simulink model "ctc_sim"  (R2019b)
settings: Solver=VariableStepAuto  StartTime=0.0  StopTime=T  FixedStep=0.001  MaxStep=0.01  RelTol=1e-3
values from neighbouring files (symbols this model uses):
  bsc = 17    [model_data.m]
  d_r = 0.01*ones(6,1)    [model_data.m]
  Fi_b_z = [0;2/3;4/3;1/3;3/3;5/3]*pi    [model_data.m]
  ksc = 1.79e5    (= 179000)    [model_data.m]
  l_r = 0.36*ones(6,1)    [model_data.m]
  linderiv = 1    [linearize_plant.m]    (also in model_data.m = 0)
  O_lb = [0;0;0;0;0;0]    [model_data.m]
  q_d = [0.523598775598 0.523598775598 -0.713724378945 0.125327831168 0.281034901503 -0.675131532937 0.281034901503 -0.675131532937 0.523598775598 0.523598775598 -0.713724378945 0.125327831168 ... (12582 elements, 18x699)]    [ik.mat]
  qt_d = [0 0 0 0 0 0 0 0 0 0 0 0 ... (12582 elements, 18x699)]    [ik.mat]
  qtt_d = [6.28830321148e-13 -2.00728322852e-12 2.02267832113e-12 3.08516978789e-12 -6.72993285032e-12 -1.57655277981e-14 7.06082029373e-13 -2.74630882455e-12 2.48904434051e-12 -1.77039226713e-12 -3.57348306345e-12 -1.6692908872e-12 ... (12582 elements, 18x699)]    [ik.mat]
  s = out_ctc.s    [ctc_run.m]
  s_0 = s_d(:,:,1)    [ctc_run.m]    (also in iff_run.m)
  t_d = [0 0.01 0.02 0.03 0.04 0.05 0.06 0.07 0.08 0.09 0.1 0.11 ... (699 elements, 1x699)]    [ik.mat]
  v_0 = v_d(:,:,1)    [ctc_run.m]    (also in iff_run.m)
  w_lb = 0.195    [model_data.m]
  W_lb = 0.205    [model_data.m]
  w_ub = 0.195    [model_data.m]
  W_ub = 0.205    [model_data.m]
  X = fminsearch(fun,X0,opts)    [iff_diag_altopt.m]    (also in iff_single_altopt.m)
undefined symbols (not defined in the file or in its folder): Kd, Ki, Kp, Y, Z
libraries: nesl_utility x260, sm_lib x204, dspindex x30, simulink_extras x18
(part 12 of 13)

== system ctc_sim/dynamic model/rods + bases/rod 6 ==
  Mux1 : Mux  Inputs=6
  Mux2 : Mux  Inputs=6
  "O_r -> G_r" : sm_lib/Frames and Transforms/Rigid Transform  TranslationMethod=StandardAxis  TranslationStandardOffset=l_r(r)/2  TranslationLengthUnit=m  TranslationStandardAxis=-Z  TranslationCartesianOffset=[0 0 0]  TranslationROffset=0  TranslationROffsetUnits=m  TranslationZOffset=0  TranslationZOffsetUnits=m  TranslationThetaOffset=0  TranslationThetaOffsetUnits=deg  RotationMethod=None  RotationAngleUnits=deg  RotationStandardAxis=+Z  RotationAngle=0.0  RotationArbitraryAxis=[0 0 1]  FollAlignAxisA=+X  BaseAlignAxisA=+Y  FollAlignAxisB=+Y  BaseAlignAxisB=+Z  RotationSequenceAxes=FollowerAxes  RotationSequence=XYX  RotationSequenceAngles=[0 0 0]  RotationSequenceAnglesUnits=deg  RotationMatrix=[1 0 0; 0 1 0; 0 0 1]
  "O_r -> H_r" : sm_lib/Frames and Transforms/Rigid Transform  TranslationMethod=StandardAxis  TranslationStandardOffset=l_r(r)/2  TranslationLengthUnit=m  TranslationStandardAxis=+Z  TranslationCartesianOffset=[0 0 0]  TranslationROffset=0  TranslationROffsetUnits=m  TranslationZOffset=0  TranslationZOffsetUnits=m  TranslationThetaOffset=0  TranslationThetaOffsetUnits=deg  RotationMethod=None  RotationAngleUnits=deg  RotationStandardAxis=+Z  RotationAngle=0.0  RotationArbitraryAxis=[0 0 1]  FollAlignAxisA=+X  BaseAlignAxisA=+Y  FollAlignAxisB=+Y  BaseAlignAxisB=+Z  RotationSequenceAxes=FollowerAxes  RotationSequence=XYX  RotationSequenceAngles=[0 0 0]  RotationSequenceAnglesUnits=deg  RotationMatrix=[1 0 0; 0 1 0; 0 0 1]
  PS-Simulink Converter : nesl_utility/PS-Simulink Converter  PhysicalDomain=network_engine_domain  SubClassName=ps_output  LeftPortType=input  RightPortType=output  PseudoPeriodic=off  Frequencies=[]  Unit=m  AffineConversion=off
  PS-Simulink Converter1 : nesl_utility/PS-Simulink Converter  PhysicalDomain=network_engine_domain  SubClassName=ps_output  LeftPortType=input  RightPortType=output  PseudoPeriodic=off  Frequencies=[]  Unit=m  AffineConversion=off
  PS-Simulink Converter10 : nesl_utility/PS-Simulink Converter  PhysicalDomain=network_engine_domain  SubClassName=ps_output  LeftPortType=input  RightPortType=output  PseudoPeriodic=off  Frequencies=[]  Unit=m/s  AffineConversion=off
  PS-Simulink Converter11 : nesl_utility/PS-Simulink Converter  PhysicalDomain=network_engine_domain  SubClassName=ps_output  LeftPortType=input  RightPortType=output  PseudoPeriodic=off  Frequencies=[]  Unit=rad/s  AffineConversion=off
  PS-Simulink Converter12 : nesl_utility/PS-Simulink Converter  PhysicalDomain=network_engine_domain  SubClassName=ps_output  LeftPortType=input  RightPortType=output  PseudoPeriodic=off  Frequencies=[]  Unit=rad/s  AffineConversion=off
  PS-Simulink Converter13 : nesl_utility/PS-Simulink Converter  PhysicalDomain=network_engine_domain  SubClassName=ps_output  LeftPortType=input  RightPortType=output  PseudoPeriodic=off  Frequencies=[]  Unit=rad/s  AffineConversion=off
  PS-Simulink Converter2 : nesl_utility/PS-Simulink Converter  PhysicalDomain=network_engine_domain  SubClassName=ps_output  LeftPortType=input  RightPortType=output  PseudoPeriodic=off  Frequencies=[]  Unit=m  AffineConversion=off
  PS-Simulink Converter3 : nesl_utility/PS-Simulink Converter  PhysicalDomain=network_engine_domain  SubClassName=ps_output  LeftPortType=input  RightPortType=output  PseudoPeriodic=off  Frequencies=[]  Unit=rad  AffineConversion=off
  PS-Simulink Converter5 : nesl_utility/PS-Simulink Converter  PhysicalDomain=network_engine_domain  SubClassName=ps_output  LeftPortType=input  RightPortType=output  PseudoPeriodic=off  Frequencies=[]  Unit=rad  AffineConversion=off
  PS-Simulink Converter7 : nesl_utility/PS-Simulink Converter  PhysicalDomain=network_engine_domain  SubClassName=ps_output  LeftPortType=input  RightPortType=output  PseudoPeriodic=off  Frequencies=[]  Unit=rad  AffineConversion=off
  PS-Simulink Converter8 : nesl_utility/PS-Simulink Converter  PhysicalDomain=network_engine_domain  SubClassName=ps_output  LeftPortType=input  RightPortType=output  PseudoPeriodic=off  Frequencies=[]  Unit=m/s  AffineConversion=off
  PS-Simulink Converter9 : nesl_utility/PS-Simulink Converter  PhysicalDomain=network_engine_domain  SubClassName=ps_output  LeftPortType=input  RightPortType=output  PseudoPeriodic=off  Frequencies=[]  Unit=m/s  AffineConversion=off
  body_r : sm_lib/Body Elements/Cylindrical Solid  GraphicAmbientColor=[0.15 0.15 0.15 1.0]  BasedOnType=Density  CenterOfMass=[0 0 0]  CenterOfMassUnits=m  GraphicDiffuseColor=model_color  CylinderLength=l_r(r)  CylinderLengthUnits=m  CylinderRadius=d_r(r)/2  CylinderRadiusUnits=m  Density=Ro_r  DensityUnits=kg/m^3  DoExposeReferenceFrame=on  GraphicEmissiveColor=[0.0 0.0 0.0 1.0]  ExportEntireGeometry=off  SerializedFrames=<Frames/>  MarkerShape=Sphere  MarkerSize=10  GraphicType=FromGeometry  InertiaType=CalculateFromGeometry  Mass=1  MassUnits=kg  MomentsOfInertia=[1 1 1]  MomentsOfInertiaUnits=kg*m^2  GraphicOpacity=model_opacity  ProductsOfInertia=[0 0 0]  ProductsOfInertiaUnits=kg*m^2  GraphicShininess=75  GraphicSpecularColor=[0.5 0.5 0.5 1.0]  GraphicVisPropType=SimpleVisualProperties
  "wf -> O_r" : sm_lib/Joints/Bushing Joint  JointMode=Normal  SenseConstraintForce=off  SenseConstraintForceX=off  SenseConstraintForceY=off  SenseConstraintForceZ=off  SenseConstraintTorque=off  SenseConstraintTorqueX=off  SenseConstraintTorqueY=off  SenseConstraintTorqueZ=off  SenseTotalForce=off  SenseTotalForceX=off  SenseTotalForceY=off  SenseTotalForceZ=off  SenseTotalTorque=off  SenseTotalTorqueX=off  SenseTotalTorqueY=off  SenseTotalTorqueZ=off  CompositeWrenchDir=FollowerOnBase  CompositeWrenchFrame=BaseFrame  PxEquilibriumPosition=0  PxEquilibriumPositionUnits=m  PxSpringStiffness=0  PxSpringStiffnessUnits=N/m  PxDampingCoefficient=0  PxDampingCoefficientUnits=N/(m/s)  PxTorqueActuationMode=NoTorque  PxMotionActuationMode=ComputedMotion  PxSensePosition=on  PxSenseVelocity=on  PxSenseAcceleration=off  PxSenseTorqueForce=off  PxSenseLowerLimitTorqueForce=off  PxSenseUpperLimitTorqueForce=off  PxLowerLimitSpecify=off  PxLowerLimitBound=-1  PxLowerLimitBoundUnits=m  PxLowerLimitStiffness=1e6  PxLowerLimitStiffnessUnits=N/m  PxLowerLimitDamping=1e3  PxLowerLimitDampingUnits=N/(m/s)  PxLowerLimitTransitionRegionWidth=1e-4  PxLowerLimitTransitionRegionWidthUnits=m  PxUpperLimitSpecify=off  PxUpperLimitBound=1  PxUpperLimitBoundUnits=m  PxUpperLimitStiffness=1e6  PxUpperLimitStiffnessUnits=N/m  PxUpperLimitDamping=1e3  PxUpperLimitDampingUnits=N/(m/s)  PxUpperLimitTransitionRegionWidth=1e-4  PxUpperLimitTransitionRegionWidthUnits=m  PxPositionTargetSpecify=on  PxPositionTargetPriority=High  PxPositionTargetValue=s_r_0(1,r)  PxPositionTargetValueUnits=m  PxVelocityTargetSpecify=on  PxVelocityTargetPriority=High  PxVelocityTargetValue=v_r_0(1,r)  PxVelocityTargetValueUnits=m/s  PyEquilibriumPosition=0  PyEquilibriumPositionUnits=m  PySpringStiffness=0  PySpringStiffnessUnits=N/m  PyDampingCoefficient=0  PyDampingCoefficientUnits=N/(m/s)  PyTorqueActuationMode=NoTorque  PyMotionActuationMode=ComputedMotion  PySensePosition=on  PySenseVelocity=on  PySenseAcceleration=off  PySenseTorqueForce=off  PySenseLowerLimitTorqueForce=off  PySenseUpperLimitTorqueForce=off  PyLowerLimitSpecify=off  PyLowerLimitBound=-1  PyLowerLimitBoundUnits=m  PyLowerLimitStiffness=1e6  PyLowerLimitStiffnessUnits=N/m  PyLowerLimitDamping=1e3  PyLowerLimitDampingUnits=N/(m/s)  PyLowerLimitTransitionRegionWidth=1e-4  PyLowerLimitTransitionRegionWidthUnits=m  PyUpperLimitSpecify=off  PyUpperLimitBound=1  PyUpperLimitBoundUnits=m  PyUpperLimitStiffness=1e6  PyUpperLimitStiffnessUnits=N/m  PyUpperLimitDamping=1e3  PyUpperLimitDampingUnits=N/(m/s)  PyUpperLimitTransitionRegionWidth=1e-4  PyUpperLimitTransitionRegionWidthUnits=m  PyPositionTargetSpecify=on  PyPositionTargetPriority=High  PyPositionTargetValue=s_r_0(2,r)  PyPositionTargetValueUnits=m  PyVelocityTargetSpecify=on  PyVelocityTargetPriority=High  PyVelocityTargetValue=v_r_0(2,r)  PyVelocityTargetValueUnits=m/s  PzEquilibriumPosition=0  PzEquilibriumPositionUnits=m  PzSpringStiffness=0  PzSpringStiffnessUnits=N/m  PzDampingCoefficient=0  PzDampingCoefficientUnits=N/(m/s)  PzTorqueActuationMode=NoTorque  PzMotionActuationMode=ComputedMotion  PzSensePosition=on  PzSenseVelocity=on  PzSenseAcceleration=off  PzSenseTorqueForce=off  PzSenseLowerLimitTorqueForce=off  PzSenseUpperLimitTorqueForce=off  PzLowerLimitSpecify=off  PzLowerLimitBound=-1  PzLowerLimitBoundUnits=m  PzLowerLimitStiffness=1e6  PzLowerLimitStiffnessUnits=N/m  PzLowerLimitDamping=1e3  PzLowerLimitDampingUnits=N/(m/s)  PzLowerLimitTransitionRegionWidth=1e-4  PzLowerLimitTransitionRegionWidthUnits=m  PzUpperLimitSpecify=off  PzUpperLimitBound=1  PzUpperLimitBoundUnits=m  PzUpperLimitStiffness=1e6  PzUpperLimitStiffnessUnits=N/m  PzUpperLimitDamping=1e3  PzUpperLimitDampingUnits=N/(m/s)  PzUpperLimitTransitionRegionWidth=1e-4  PzUpperLimitTransitionRegionWidthUnits=m  PzPositionTargetSpecify=on  PzPositionTargetPriority=High  PzPositionTargetValue=s_r_0(3,r)  PzPositionTargetValueUnits=m  PzVelocityTargetSpecify=on  PzVelocityTargetPriority=High  PzVelocityTargetValue=v_r_0(3,r)  PzVelocityTargetValueUnits=m/s  RxEquilibriumPosition=0  RxEquilibriumPositionUnits=deg  RxSpringStiffness=0  RxSpringStiffnessUnits=N*m/deg  RxDampingCoefficient=0  RxDampingCoefficientUnits=N*m/(deg/s)  RxTorqueActuationMode=NoTorque  RxMotionActuationMode=ComputedMotion  RxSensePosition=on  RxSenseVelocity=on  RxSenseAcceleration=off  RxSenseTorqueForce=off  RxSenseLowerLimitTorqueForce=off  RxSenseUpperLimitTorqueForce=off  RxLowerLimitSpecify=off  RxLowerLimitBound=-90  RxLowerLimitBoundUnits=deg  RxLowerLimitStiffness=1e4  RxLowerLimitStiffnessUnits=N*m/deg  RxLowerLimitDamping=10  RxLowerLimitDampingUnits=N*m/(deg/s)  RxLowerLimitTransitionRegionWidth=0.1  RxLowerLimitTransitionRegionWidthUnits=deg  RxUpperLimitSpecify=off  RxUpperLimitBound=90  RxUpperLimitBoundUnits=deg  RxUpperLimitStiffness=1e4  RxUpperLimitStiffnessUnits=N*m/deg  RxUpperLimitDamping=10  RxUpperLimitDampingUnits=N*m/(deg/s)  RxUpperLimitTransitionRegionWidth=0.1  RxUpperLimitTransitionRegionWidthUnits=deg  RxPositionTargetSpecify=on  RxPositionTargetPriority=High  RxPositionTargetValue=s_r_0(4,r)  RxPositionTargetValueUnits=rad  RxVelocityTargetSpecify=on  RxVelocityTargetPriority=High  RxVelocityTargetValue=v_r_0(4,r)  RxVelocityTargetValueUnits=rad/s  RyEquilibriumPosition=0  RyEquilibriumPositionUnits=deg  RySpringStiffness=0  RySpringStiffnessUnits=N*m/deg  RyDampingCoefficient=0  RyDampingCoefficientUnits=N*m/(deg/s)  RyTorqueActuationMode=NoTorque  RyMotionActuationMode=ComputedMotion  RySensePosition=on  RySenseVelocity=on  RySenseAcceleration=off  RySenseTorqueForce=off  RySenseLowerLimitTorqueForce=off  RySenseUpperLimitTorqueForce=off  RyLowerLimitSpecify=off  RyLowerLimitBound=-90  RyLowerLimitBoundUnits=deg  RyLowerLimitStiffness=1e4  RyLowerLimitStiffnessUnits=N*m/deg  RyLowerLimitDamping=10  RyLowerLimitDampingUnits=N*m/(deg/s)  RyLowerLimitTransitionRegionWidth=0.1  RyLowerLimitTransitionRegionWidthUnits=deg  RyUpperLimitSpecify=off  RyUpperLimitBound=90  RyUpperLimitBoundUnits=deg  RyUpperLimitStiffness=1e4  RyUpperLimitStiffnessUnits=N*m/deg  RyUpperLimitDamping=10  RyUpperLimitDampingUnits=N*m/(deg/s)  RyUpperLimitTransitionRegionWidth=0.1  RyUpperLimitTransitionRegionWidthUnits=deg  RyPositionTargetSpecify=on  RyPositionTargetPriority=High  RyPositionTargetValue=s_r_0(5,r)  RyPositionTargetValueUnits=rad  RyVelocityTargetSpecify=on  RyVelocityTargetPriority=High  RyVelocityTargetValue=v_r_0(5,r)  RyVelocityTargetValueUnits=rad/s  RzEquilibriumPosition=0  RzEquilibriumPositionUnits=deg  RzSpringStiffness=0  RzSpringStiffnessUnits=N*m/deg  RzDampingCoefficient=0  RzDampingCoefficientUnits=N*m/(deg/s)  RzTorqueActuationMode=NoTorque  RzMotionActuationMode=ComputedMotion  RzSensePosition=on  RzSenseVelocity=on  RzSenseAcceleration=off  RzSenseTorqueForce=off  RzSenseLowerLimitTorqueForce=off  RzSenseUpperLimitTorqueForce=off  RzLowerLimitSpecify=off  RzLowerLimitBound=-90  RzLowerLimitBoundUnits=deg  RzLowerLimitStiffness=1e4  RzLowerLimitStiffnessUnits=N*m/deg  RzLowerLimitDamping=10  RzLowerLimitDampingUnits=N*m/(deg/s)  RzLowerLimitTransitionRegionWidth=0.1  RzLowerLimitTransitionRegionWidthUnits=deg  RzUpperLimitSpecify=off  RzUpperLimitBound=90  RzUpperLimitBoundUnits=deg  RzUpperLimitStiffness=1e4  RzUpperLimitStiffnessUnits=N*m/deg  RzUpperLimitDamping=10  RzUpperLimitDampingUnits=N*m/(deg/s)  RzUpperLimitTransitionRegionWidth=0.1  RzUpperLimitTransitionRegionWidthUnits=deg  RzPositionTargetSpecify=on  RzPositionTargetPriority=High  RzPositionTargetValue=s_r_0(6,r)  RzPositionTargetValueUnits=rad  RzVelocityTargetSpecify=on  RzVelocityTargetPriority=High  RzVelocityTargetValue=v_r_0(6,r)  RzVelocityTargetValueUnits=rad/s
      settings: SourceProductName=Simscape Multibody
  wf : PMIOPort  Side=Left
  G_r : PMIOPort  Port=2  Side=Right
  H_r : PMIOPort  Port=3  Side=Left
  s_r : Outport
  v_r : Outport  Port=2
  wires:
  Mux1/1 -> s_r/1
  PS-Simulink Converter/1 -> Mux1/1
  PS-Simulink Converter1/1 -> Mux1/2
  PS-Simulink Converter2/1 -> Mux1/3
  PS-Simulink Converter3/1 -> Mux1/4
  PS-Simulink Converter5/1 -> Mux1/5
  PS-Simulink Converter7/1 -> Mux1/6
  Mux2/1 -> v_r/1
  PS-Simulink Converter8/1 -> Mux2/1
  PS-Simulink Converter9/1 -> Mux2/2
  PS-Simulink Converter10/1 -> Mux2/3
  PS-Simulink Converter11/1 -> Mux2/4
  PS-Simulink Converter12/1 -> Mux2/5
  PS-Simulink Converter13/1 -> Mux2/6
  connections:
  "wf -> O_r"/LConn1 -- wf/RConn1
  "O_r -> G_r"/LConn1 -- body_r/RConn1 -- "wf -> O_r"/RConn1 -- "O_r -> H_r"/LConn1
  H_r/RConn1 -- "O_r -> H_r"/RConn1
  G_r/RConn1 -- "O_r -> G_r"/RConn1
  PS-Simulink Converter/LConn1 -- "wf -> O_r"/RConn2
  PS-Simulink Converter1/LConn1 -- "wf -> O_r"/RConn4
  PS-Simulink Converter2/LConn1 -- "wf -> O_r"/RConn6
  "wf -> O_r"/RConn8 -- PS-Simulink Converter3/LConn1
  PS-Simulink Converter8/LConn1 -- "wf -> O_r"/RConn3
  PS-Simulink Converter9/LConn1 -- "wf -> O_r"/RConn5
  PS-Simulink Converter10/LConn1 -- "wf -> O_r"/RConn7
  PS-Simulink Converter11/LConn1 -- "wf -> O_r"/RConn9
  PS-Simulink Converter13/LConn1 -- "wf -> O_r"/RConn13
  "wf -> O_r"/RConn12 -- PS-Simulink Converter7/LConn1
  PS-Simulink Converter12/LConn1 -- "wf -> O_r"/RConn11
  "wf -> O_r"/RConn10 -- PS-Simulink Converter5/LConn1

== system ctc_sim/dynamic model/rods + bases/upper base ==
  Mux1 : Mux  Inputs=6
  Mux2 : Mux  Inputs=6
  "O_ub -> H_4" : Subsystem
  "O_ub -> H_5" : Subsystem
  "O_ub -> H_6" : Subsystem
  PS-Simulink Converter : nesl_utility/PS-Simulink Converter  PhysicalDomain=network_engine_domain  SubClassName=ps_output  LeftPortType=input  RightPortType=output  PseudoPeriodic=off  Frequencies=[]  Unit=m  AffineConversion=off
  PS-Simulink Converter10 : nesl_utility/PS-Simulink Converter  PhysicalDomain=network_engine_domain  SubClassName=ps_output  LeftPortType=input  RightPortType=output  PseudoPeriodic=off  Frequencies=[]  Unit=rad  AffineConversion=off
  PS-Simulink Converter12 : nesl_utility/PS-Simulink Converter  PhysicalDomain=network_engine_domain  SubClassName=ps_output  LeftPortType=input  RightPortType=output  PseudoPeriodic=off  Frequencies=[]  Unit=m/s  AffineConversion=off
  PS-Simulink Converter13 : nesl_utility/PS-Simulink Converter  PhysicalDomain=network_engine_domain  SubClassName=ps_output  LeftPortType=input  RightPortType=output  PseudoPeriodic=off  Frequencies=[]  Unit=m/s  AffineConversion=off
  PS-Simulink Converter14 : nesl_utility/PS-Simulink Converter  PhysicalDomain=network_engine_domain  SubClassName=ps_output  LeftPortType=input  RightPortType=output  PseudoPeriodic=off  Frequencies=[]  Unit=m/s  AffineConversion=off
  PS-Simulink Converter15 : nesl_utility/PS-Simulink Converter  PhysicalDomain=network_engine_domain  SubClassName=ps_output  LeftPortType=input  RightPortType=output  PseudoPeriodic=off  Frequencies=[]  Unit=rad/s  AffineConversion=off
  PS-Simulink Converter16 : nesl_utility/PS-Simulink Converter  PhysicalDomain=network_engine_domain  SubClassName=ps_output  LeftPortType=input  RightPortType=output  PseudoPeriodic=off  Frequencies=[]  Unit=rad/s  AffineConversion=off
  PS-Simulink Converter17 : nesl_utility/PS-Simulink Converter  PhysicalDomain=network_engine_domain  SubClassName=ps_output  LeftPortType=input  RightPortType=output  PseudoPeriodic=off  Frequencies=[]  Unit=rad/s  AffineConversion=off
  PS-Simulink Converter2 : nesl_utility/PS-Simulink Converter  PhysicalDomain=network_engine_domain  SubClassName=ps_output  LeftPortType=input  RightPortType=output  PseudoPeriodic=off  Frequencies=[]  Unit=m  AffineConversion=off
  PS-Simulink Converter4 : nesl_utility/PS-Simulink Converter  PhysicalDomain=network_engine_domain  SubClassName=ps_output  LeftPortType=input  RightPortType=output  PseudoPeriodic=off  Frequencies=[]  Unit=m  AffineConversion=off
  PS-Simulink Converter6 : nesl_utility/PS-Simulink Converter  PhysicalDomain=network_engine_domain  SubClassName=ps_output  LeftPortType=input  RightPortType=output  PseudoPeriodic=off  Frequencies=[]  Unit=rad  AffineConversion=off
  PS-Simulink Converter8 : nesl_utility/PS-Simulink Converter  PhysicalDomain=network_engine_domain  SubClassName=ps_output  LeftPortType=input  RightPortType=output  PseudoPeriodic=off  Frequencies=[]  Unit=rad  AffineConversion=off
  body_ub : sm_lib/Body Elements/Extruded Solid  GraphicAmbientColor=[0.15 0.15 0.15 1.0]  BasedOnType=Density  CenterOfMass=[0 0 0]  CenterOfMassUnits=m  GraphicDiffuseColor=model_color  ExtrusionCrossSection=[1 1; -1 1; -1 -1; 1 -1]  ExtrusionCrossSectionUnits=m  Density=Ro_ub  DensityUnits=kg/m^3  DoExposeReferenceFrame=on  GraphicEmissiveColor=[0.0 0.0 0.0 1.0]  ExportEntireGeometry=off  ExtrusionLength=t_ub  ExtrusionLengthUnits=m  ExtrusionType=Regular  SerializedFrames=<Frames/>  MarkerShape=Sphere  MarkerSize=10  GraphicType=FromGeometry  InertiaType=CalculateFromGeometry  Mass=1  MassUnits=kg  MomentsOfInertia=[1 1 1]  MomentsOfInertiaUnits=kg*m^2  PolygonNumSides=6  GraphicOpacity=model_opacity  PolygonOuterRadius=(W_ub/2)/cosd(30)  PolygonOuterRadiusUnits=m  ProductsOfInertia=[0 0 0]  ProductsOfInertiaUnits=kg*m^2  GraphicShininess=75  GraphicSpecularColor=[0.5 0.5 0.5 1.0]  GraphicVisPropType=SimpleVisualProperties
      settings: SourceProductName=Simscape Multibody
  "wf -> O_ub" : sm_lib/Joints/Bushing Joint  JointMode=Normal  SenseConstraintForce=off  SenseConstraintForceX=off  SenseConstraintForceY=off  SenseConstraintForceZ=off  SenseConstraintTorque=off  SenseConstraintTorqueX=off  SenseConstraintTorqueY=off  SenseConstraintTorqueZ=off  SenseTotalForce=off  SenseTotalForceX=off  SenseTotalForceY=off  SenseTotalForceZ=off  SenseTotalTorque=off  SenseTotalTorqueX=off  SenseTotalTorqueY=off  SenseTotalTorqueZ=off  CompositeWrenchDir=FollowerOnBase  CompositeWrenchFrame=BaseFrame  PxEquilibriumPosition=0  PxEquilibriumPositionUnits=m  PxSpringStiffness=0  PxSpringStiffnessUnits=N/m  PxDampingCoefficient=0  PxDampingCoefficientUnits=N/(m/s)  PxTorqueActuationMode=NoTorque  PxMotionActuationMode=ComputedMotion  PxSensePosition=on  PxSenseVelocity=on  PxSenseAcceleration=off  PxSenseTorqueForce=off  PxSenseLowerLimitTorqueForce=off  PxSenseUpperLimitTorqueForce=off  PxLowerLimitSpecify=off  PxLowerLimitBound=-1  PxLowerLimitBoundUnits=m  PxLowerLimitStiffness=1e6  PxLowerLimitStiffnessUnits=N/m  PxLowerLimitDamping=1e3  PxLowerLimitDampingUnits=N/(m/s)  PxLowerLimitTransitionRegionWidth=1e-4  PxLowerLimitTransitionRegionWidthUnits=m  PxUpperLimitSpecify=off  PxUpperLimitBound=1  PxUpperLimitBoundUnits=m  PxUpperLimitStiffness=1e6  PxUpperLimitStiffnessUnits=N/m  PxUpperLimitDamping=1e3  PxUpperLimitDampingUnits=N/(m/s)  PxUpperLimitTransitionRegionWidth=1e-4  PxUpperLimitTransitionRegionWidthUnits=m  PxPositionTargetSpecify=on  PxPositionTargetPriority=High  PxPositionTargetValue=s_ub_0(1,1)  PxPositionTargetValueUnits=m  PxVelocityTargetSpecify=on  PxVelocityTargetPriority=High  PxVelocityTargetValue=v_ub_0(1,1)  PxVelocityTargetValueUnits=m/s  PyEquilibriumPosition=0  PyEquilibriumPositionUnits=m  PySpringStiffness=0  PySpringStiffnessUnits=N/m  PyDampingCoefficient=0  PyDampingCoefficientUnits=N/(m/s)  PyTorqueActuationMode=NoTorque  PyMotionActuationMode=ComputedMotion  PySensePosition=on  PySenseVelocity=on  PySenseAcceleration=off  PySenseTorqueForce=off  PySenseLowerLimitTorqueForce=off  PySenseUpperLimitTorqueForce=off  PyLowerLimitSpecify=off  PyLowerLimitBound=-1  PyLowerLimitBoundUnits=m  PyLowerLimitStiffness=1e6  PyLowerLimitStiffnessUnits=N/m  PyLowerLimitDamping=1e3  PyLowerLimitDampingUnits=N/(m/s)  PyLowerLimitTransitionRegionWidth=1e-4  PyLowerLimitTransitionRegionWidthUnits=m  PyUpperLimitSpecify=off  PyUpperLimitBound=1  PyUpperLimitBoundUnits=m  PyUpperLimitStiffness=1e6  PyUpperLimitStiffnessUnits=N/m  PyUpperLimitDamping=1e3  PyUpperLimitDampingUnits=N/(m/s)  PyUpperLimitTransitionRegionWidth=1e-4  PyUpperLimitTransitionRegionWidthUnits=m  PyPositionTargetSpecify=on  PyPositionTargetPriority=High  PyPositionTargetValue=s_ub_0(2,1)  PyPositionTargetValueUnits=m  PyVelocityTargetSpecify=on  PyVelocityTargetPriority=High  PyVelocityTargetValue=v_ub_0(2,1)  PyVelocityTargetValueUnits=m/s  PzEquilibriumPosition=0  PzEquilibriumPositionUnits=m  PzSpringStiffness=0  PzSpringStiffnessUnits=N/m  PzDampingCoefficient=0  PzDampingCoefficientUnits=N/(m/s)  PzTorqueActuationMode=NoTorque  PzMotionActuationMode=ComputedMotion  PzSensePosition=on  PzSenseVelocity=on  PzSenseAcceleration=off  PzSenseTorqueForce=off  PzSenseLowerLimitTorqueForce=off  PzSenseUpperLimitTorqueForce=off  PzLowerLimitSpecify=off  PzLowerLimitBound=-1  PzLowerLimitBoundUnits=m  PzLowerLimitStiffness=1e6  PzLowerLimitStiffnessUnits=N/m  PzLowerLimitDamping=1e3  PzLowerLimitDampingUnits=N/(m/s)  PzLowerLimitTransitionRegionWidth=1e-4  PzLowerLimitTransitionRegionWidthUnits=m  PzUpperLimitSpecify=off  PzUpperLimitBound=1  PzUpperLimitBoundUnits=m  PzUpperLimitStiffness=1e6  PzUpperLimitStiffnessUnits=N/m  PzUpperLimitDamping=1e3  PzUpperLimitDampingUnits=N/(m/s)  PzUpperLimitTransitionRegionWidth=1e-4  PzUpperLimitTransitionRegionWidthUnits=m  PzPositionTargetSpecify=on  PzPositionTargetPriority=High  PzPositionTargetValue=s_ub_0(3,1)  PzPositionTargetValueUnits=m  PzVelocityTargetSpecify=on  PzVelocityTargetPriority=High  PzVelocityTargetValue=v_ub_0(3,1)  PzVelocityTargetValueUnits=m/s  RxEquilibriumPosition=0  RxEquilibriumPositionUnits=deg  RxSpringStiffness=0  RxSpringStiffnessUnits=N*m/deg  RxDampingCoefficient=0  RxDampingCoefficientUnits=N*m/(deg/s)  RxTorqueActuationMode=NoTorque  RxMotionActuationMode=ComputedMotion  RxSensePosition=on  RxSenseVelocity=on  RxSenseAcceleration=off  RxSenseTorqueForce=off  RxSenseLowerLimitTorqueForce=off  RxSenseUpperLimitTorqueForce=off  RxLowerLimitSpecify=off  RxLowerLimitBound=-90  RxLowerLimitBoundUnits=deg  RxLowerLimitStiffness=1e4  RxLowerLimitStiffnessUnits=N*m/deg  RxLowerLimitDamping=10  RxLowerLimitDampingUnits=N*m/(deg/s)  RxLowerLimitTransitionRegionWidth=0.1  RxLowerLimitTransitionRegionWidthUnits=deg  RxUpperLimitSpecify=off  RxUpperLimitBound=90  RxUpperLimitBoundUnits=deg  RxUpperLimitStiffness=1e4  RxUpperLimitStiffnessUnits=N*m/deg  RxUpperLimitDamping=10  RxUpperLimitDampingUnits=N*m/(deg/s)  RxUpperLimitTransitionRegionWidth=0.1  RxUpperLimitTransitionRegionWidthUnits=deg  RxPositionTargetSpecify=on  RxPositionTargetPriority=High  RxPositionTargetValue=s_ub_0(4,1)  RxPositionTargetValueUnits=rad  RxVelocityTargetSpecify=on  RxVelocityTargetPriority=High  RxVelocityTargetValue=v_ub_0(4,1)  RxVelocityTargetValueUnits=rad/s  RyEquilibriumPosition=0  RyEquilibriumPositionUnits=deg  RySpringStiffness=0  RySpringStiffnessUnits=N*m/deg  RyDampingCoefficient=0  RyDampingCoefficientUnits=N*m/(deg/s)  RyTorqueActuationMode=NoTorque  RyMotionActuationMode=ComputedMotion  RySensePosition=on  RySenseVelocity=on  RySenseAcceleration=off  RySenseTorqueForce=off  RySenseLowerLimitTorqueForce=off  RySenseUpperLimitTorqueForce=off  RyLowerLimitSpecify=off  RyLowerLimitBound=-90  RyLowerLimitBoundUnits=deg  RyLowerLimitStiffness=1e4  RyLowerLimitStiffnessUnits=N*m/deg  RyLowerLimitDamping=10  RyLowerLimitDampingUnits=N*m/(deg/s)  RyLowerLimitTransitionRegionWidth=0.1  RyLowerLimitTransitionRegionWidthUnits=deg  RyUpperLimitSpecify=off  RyUpperLimitBound=90  RyUpperLimitBoundUnits=deg  RyUpperLimitStiffness=1e4  RyUpperLimitStiffnessUnits=N*m/deg  RyUpperLimitDamping=10  RyUpperLimitDampingUnits=N*m/(deg/s)  RyUpperLimitTransitionRegionWidth=0.1  RyUpperLimitTransitionRegionWidthUnits=deg  RyPositionTargetSpecify=on  RyPositionTargetPriority=High  RyPositionTargetValue=s_ub_0(5,1)  RyPositionTargetValueUnits=rad  RyVelocityTargetSpecify=on  RyVelocityTargetPriority=High  RyVelocityTargetValue=v_ub_0(5,1)  RyVelocityTargetValueUnits=rad/s  RzEquilibriumPosition=0  RzEquilibriumPositionUnits=deg  RzSpringStiffness=0  RzSpringStiffnessUnits=N*m/deg  RzDampingCoefficient=0  RzDampingCoefficientUnits=N*m/(deg/s)  RzTorqueActuationMode=NoTorque  RzMotionActuationMode=ComputedMotion  RzSensePosition=on  RzSenseVelocity=on  RzSenseAcceleration=off  RzSenseTorqueForce=off  RzSenseLowerLimitTorqueForce=off  RzSenseUpperLimitTorqueForce=off  RzLowerLimitSpecify=off  RzLowerLimitBound=-90  RzLowerLimitBoundUnits=deg  RzLowerLimitStiffness=1e4  RzLowerLimitStiffnessUnits=N*m/deg  RzLowerLimitDamping=10  RzLowerLimitDampingUnits=N*m/(deg/s)  RzLowerLimitTransitionRegionWidth=0.1  RzLowerLimitTransitionRegionWidthUnits=deg  RzUpperLimitSpecify=off  RzUpperLimitBound=90  RzUpperLimitBoundUnits=deg  RzUpperLimitStiffness=1e4  RzUpperLimitStiffnessUnits=N*m/deg  RzUpperLimitDamping=10  RzUpperLimitDampingUnits=N*m/(deg/s)  RzUpperLimitTransitionRegionWidth=0.1  RzUpperLimitTransitionRegionWidthUnits=deg  RzPositionTargetSpecify=on  RzPositionTargetPriority=High  RzPositionTargetValue=s_ub_0(6,1)  RzPositionTargetValueUnits=rad  RzVelocityTargetSpecify=on  RzVelocityTargetPriority=High  RzVelocityTargetValue=v_ub_0(6,1)  RzVelocityTargetValueUnits=rad/s
      settings: SourceProductName=Simscape Multibody
  H_4 : PMIOPort  Side=Right
  H_5 : PMIOPort  Port=2  Side=Right
  H_6 : PMIOPort  Port=3  Side=Right
  wf : PMIOPort  Port=4  Side=Left
  s_ub : Outport
  v_ub : Outport  Port=2
  wires:
  Mux1/1 -> s_ub/1
  PS-Simulink Converter10/1 -> Mux1/6
  PS-Simulink Converter8/1 -> Mux1/5
  PS-Simulink Converter6/1 -> Mux1/4
  PS-Simulink Converter4/1 -> Mux1/3
  PS-Simulink Converter2/1 -> Mux1/2
  PS-Simulink Converter/1 -> Mux1/1
  Mux2/1 -> v_ub/1
  PS-Simulink Converter12/1 -> Mux2/1
  PS-Simulink Converter13/1 -> Mux2/2
  PS-Simulink Converter14/1 -> Mux2/3
  PS-Simulink Converter15/1 -> Mux2/4
  PS-Simulink Converter16/1 -> Mux2/5
  PS-Simulink Converter17/1 -> Mux2/6
  connections:
  H_4/RConn1 -- "O_ub -> H_4"/RConn1
  H_5/RConn1 -- "O_ub -> H_5"/RConn1
  H_6/RConn1 -- "O_ub -> H_6"/RConn1
  "O_ub -> H_6"/LConn1 -- "wf -> O_ub"/RConn1 -- body_ub/RConn1 -- "O_ub -> H_4"/LConn1 -- "O_ub -> H_5"/LConn1
  PS-Simulink Converter/LConn1 -- "wf -> O_ub"/RConn2
  PS-Simulink Converter12/LConn1 -- "wf -> O_ub"/RConn3
  PS-Simulink Converter13/LConn1 -- "wf -> O_ub"/RConn5
  PS-Simulink Converter2/LConn1 -- "wf -> O_ub"/RConn4
  PS-Simulink Converter4/LConn1 -- "wf -> O_ub"/RConn6
  PS-Simulink Converter14/LConn1 -- "wf -> O_ub"/RConn7
  PS-Simulink Converter6/LConn1 -- "wf -> O_ub"/RConn8
  PS-Simulink Converter15/LConn1 -- "wf -> O_ub"/RConn9
  PS-Simulink Converter8/LConn1 -- "wf -> O_ub"/RConn10
  PS-Simulink Converter16/LConn1 -- "wf -> O_ub"/RConn11
  PS-Simulink Converter10/LConn1 -- "wf -> O_ub"/RConn12
  PS-Simulink Converter17/LConn1 -- "wf -> O_ub"/RConn13
  wf/RConn1 -- "wf -> O_ub"/LConn1

== system ctc_sim/dynamic model/rods + bases/world frame ==
  gravity : sm_lib/Utilities/Mechanism Configuration  UniformGravity=Constant  GravityVector=g  GravityUnits=m/s^2  LinearizationDelta=0.001
  solver config : nesl_utility/Solver Configuration  PhysicalDomain=network_engine_domain  SubClassName=solver  LeftPortType=input  RightPortType=generic  Tones=[]  Harmonics=[]  SimulateNoise=off  Profile=off  UseLocalSampling=off  EnableSwitchedLinearOptims=on  FrequencyDomain=off  UseCCode=off  RelTol=0.001  AbsTol=1e-06  MinStep=1e-09  ToWorkspace=off  RevertToSquareIcSolve=off  NumHomotopyIterations=100  PhasorMode=off  PhasorModeNumHarmonics=1  DoDC=off  ResidualTolerance=1e-09  UseLocalSolver=off  LocalSolverChoice=NE_BACKWARD_EULER_ADVANCER  LocalSolverSampleTime=0.001  DoFixedCost=off  MaxNonlinIter=3  MaxModeIter=2  LinearAlgebra=auto  EquationFormulation=NE_TIME_EF  DelaysMemoryBudget=1024  AutomaticFiltering=on  FilteringTimeConstant=0.001  PartitionStorageMethod=AS_NEEDED  PartitionMemoryBudget=1024  PartitionMethod=ROBUST
  world frame : sm_lib/Frames and Transforms/World Frame
  wf : PMIOPort  Side=Right
  connections:
  solver config/RConn1 -- world frame/RConn1 -- wf/RConn1 -- gravity/RConn1

== system ctc_sim/inverse kinematics/t -> q_d/rod 1 ==
  t : Inport
  Mux : Mux  Inputs=2
  Q_r,d,x : Lookup_n-D  NumberOfTableDimensions=1  BreakpointsForDimension1=t_d(1,:)  BreakpointsForDimension2=t_d(1,:)  Table=Q_d((r-1)*2+1,:)  InternalRulePriority=Speed  RndMeth=Simplest  InputSameDT=on
  Q_r,d,y : Lookup_n-D  NumberOfTableDimensions=1  BreakpointsForDimension1=t_d(1,:)  BreakpointsForDimension2=t_d(1,:)  Table=Q_d((r-1)*2+2,:)  InternalRulePriority=Speed  RndMeth=Simplest  InputSameDT=on
  Q_r,d : Outport
  wires:
  t/1 -> Q_r,d,y/1, Q_r,d,x/1
  Q_r,d,y/1 -> Mux/2
  Q_r,d,x/1 -> Mux/1
  Mux/1 -> Q_r,d/1

== system ctc_sim/inverse kinematics/t -> q_d/rod 2 ==
  t : Inport
  Mux : Mux  Inputs=2
  Q_r,d,x : Lookup_n-D  NumberOfTableDimensions=1  BreakpointsForDimension1=t_d(1,:)  BreakpointsForDimension2=t_d(1,:)  Table=Q_d((r-1)*2+1,:)  InternalRulePriority=Speed  RndMeth=Simplest  InputSameDT=on
  Q_r,d,y : Lookup_n-D  NumberOfTableDimensions=1  BreakpointsForDimension1=t_d(1,:)  BreakpointsForDimension2=t_d(1,:)  Table=Q_d((r-1)*2+2,:)  InternalRulePriority=Speed  RndMeth=Simplest  InputSameDT=on
  Q_r,d : Outport
  wires:
  t/1 -> Q_r,d,y/1, Q_r,d,x/1
  Q_r,d,y/1 -> Mux/2
  Q_r,d,x/1 -> Mux/1
  Mux/1 -> Q_r,d/1

== system ctc_sim/inverse kinematics/t -> q_d/rod 3 ==
  t : Inport
  Mux : Mux  Inputs=2
  Q_r,d,x : Lookup_n-D  NumberOfTableDimensions=1  BreakpointsForDimension1=t_d(1,:)  BreakpointsForDimension2=t_d(1,:)  Table=Q_d((r-1)*2+1,:)  InternalRulePriority=Speed  RndMeth=Simplest  InputSameDT=on
  Q_r,d,y : Lookup_n-D  NumberOfTableDimensions=1  BreakpointsForDimension1=t_d(1,:)  BreakpointsForDimension2=t_d(1,:)  Table=Q_d((r-1)*2+2,:)  InternalRulePriority=Speed  RndMeth=Simplest  InputSameDT=on
  Q_r,d : Outport
  wires:
  t/1 -> Q_r,d,y/1, Q_r,d,x/1
  Q_r,d,y/1 -> Mux/2
  Q_r,d,x/1 -> Mux/1
  Mux/1 -> Q_r,d/1

== system ctc_sim/inverse kinematics/t -> q_d/rod 4 ==
  t : Inport
  Mux : Mux  Inputs=2
  Q_r,d,x : Lookup_n-D  NumberOfTableDimensions=1  BreakpointsForDimension1=t_d(1,:)  BreakpointsForDimension2=t_d(1,:)  Table=Q_d((r-1)*2+1,:)  InternalRulePriority=Speed  RndMeth=Simplest  InputSameDT=on
  Q_r,d,y : Lookup_n-D  NumberOfTableDimensions=1  BreakpointsForDimension1=t_d(1,:)  BreakpointsForDimension2=t_d(1,:)  Table=Q_d((r-1)*2+2,:)  InternalRulePriority=Speed  RndMeth=Simplest  InputSameDT=on
  Q_r,d : Outport
  wires:
  t/1 -> Q_r,d,y/1, Q_r,d,x/1
  Q_r,d,y/1 -> Mux/2
  Q_r,d,x/1 -> Mux/1
  Mux/1 -> Q_r,d/1

== system ctc_sim/inverse kinematics/t -> q_d/rod 5 ==
  t : Inport
  Mux : Mux  Inputs=2
  Q_r,d,x : Lookup_n-D  NumberOfTableDimensions=1  BreakpointsForDimension1=t_d(1,:)  BreakpointsForDimension2=t_d(1,:)  Table=Q_d((r-1)*2+1,:)  InternalRulePriority=Speed  RndMeth=Simplest  InputSameDT=on
  Q_r,d,y : Lookup_n-D  NumberOfTableDimensions=1  BreakpointsForDimension1=t_d(1,:)  BreakpointsForDimension2=t_d(1,:)  Table=Q_d((r-1)*2+2,:)  InternalRulePriority=Speed  RndMeth=Simplest  InputSameDT=on
  Q_r,d : Outport
  wires:
  t/1 -> Q_r,d,y/1, Q_r,d,x/1
  Q_r,d,y/1 -> Mux/2
  Q_r,d,x/1 -> Mux/1
  Mux/1 -> Q_r,d/1

== system ctc_sim/inverse kinematics/t -> q_d/rod 6 ==
  t : Inport
  Mux : Mux  Inputs=2
  Q_r,d,x : Lookup_n-D  NumberOfTableDimensions=1  BreakpointsForDimension1=t_d(1,:)  BreakpointsForDimension2=t_d(1,:)  Table=Q_d((r-1)*2+1,:)  InternalRulePriority=Speed  RndMeth=Simplest  InputSameDT=on
  Q_r,d,y : Lookup_n-D  NumberOfTableDimensions=1  BreakpointsForDimension1=t_d(1,:)  BreakpointsForDimension2=t_d(1,:)  Table=Q_d((r-1)*2+2,:)  InternalRulePriority=Speed  RndMeth=Simplest  InputSameDT=on
  Q_r,d : Outport
  wires:
  t/1 -> Q_r,d,y/1, Q_r,d,x/1
  Q_r,d,y/1 -> Mux/2
  Q_r,d,x/1 -> Mux/1
  Mux/1 -> Q_r,d/1

== system ctc_sim/inverse kinematics/t -> q_d/upper base ==
  t : Inport
  Mux : Mux  Inputs=6
  Q_ub,d,phi_x : Lookup_n-D  NumberOfTableDimensions=1  BreakpointsForDimension1=t_d(1,:)  BreakpointsForDimension2=t_d(1,:)  Table=Q_d(16,:)  InternalRulePriority=Speed  RndMeth=Simplest  InputSameDT=on
  Q_ub,d,phi_y : Lookup_n-D  NumberOfTableDimensions=1  BreakpointsForDimension1=t_d(1,:)  BreakpointsForDimension2=t_d(1,:)  Table=Q_d(17,:)  InternalRulePriority=Speed  RndMeth=Simplest  InputSameDT=on
  Q_ub,d,phi_z : Lookup_n-D  NumberOfTableDimensions=1  BreakpointsForDimension1=t_d(1,:)  BreakpointsForDimension2=t_d(1,:)  Table=Q_d(18,:)  InternalRulePriority=Speed  RndMeth=Simplest  InputSameDT=on
  Q_ub,d,x : Lookup_n-D  NumberOfTableDimensions=1  BreakpointsForDimension1=t_d(1,:)  BreakpointsForDimension2=t_d(1,:)  Table=Q_d(13,:)  InternalRulePriority=Speed  RndMeth=Simplest  InputSameDT=on
  Q_ub,d,y : Lookup_n-D  NumberOfTableDimensions=1  BreakpointsForDimension1=t_d(1,:)  BreakpointsForDimension2=t_d(1,:)  Table=Q_d(14,:)  InternalRulePriority=Speed  RndMeth=Simplest  InputSameDT=on
  Q_ub,d,z : Lookup_n-D  NumberOfTableDimensions=1  BreakpointsForDimension1=t_d(1,:)  BreakpointsForDimension2=t_d(1,:)  Table=Q_d(15,:)  InternalRulePriority=Speed  RndMeth=Simplest  InputSameDT=on
  Q_ub,d : Outport
  wires:
  t/1 -> Q_ub,d,y/1, Q_ub,d,z/1, Q_ub,d,phi_x/1, Q_ub,d,phi_y/1, Q_ub,d,phi_z/1, Q_ub,d,x/1
  Q_ub,d,x/1 -> Mux/1
  Q_ub,d,phi_z/1 -> Mux/6
  Q_ub,d,phi_y/1 -> Mux/5
  Q_ub,d,phi_x/1 -> Mux/4
  Q_ub,d,z/1 -> Mux/3
  Q_ub,d,y/1 -> Mux/2
  Mux/1 -> Q_ub,d/1

== system ctc_sim/inverse kinematics/t -> qt_d/rod 1 ==
  t : Inport
  Mux : Mux  Inputs=2
  Q_r,d,x : Lookup_n-D  NumberOfTableDimensions=1  BreakpointsForDimension1=t_d(1,:)  BreakpointsForDimension2=t_d(1,:)  Table=Q_d((r-1)*2+1,:)  InternalRulePriority=Speed  RndMeth=Simplest  InputSameDT=on
  Q_r,d,y : Lookup_n-D  NumberOfTableDimensions=1  BreakpointsForDimension1=t_d(1,:)  BreakpointsForDimension2=t_d(1,:)  Table=Q_d((r-1)*2+2,:)  InternalRulePriority=Speed  RndMeth=Simplest  InputSameDT=on
  Q_r,d : Outport
  wires:
  t/1 -> Q_r,d,y/1, Q_r,d,x/1
  Q_r,d,y/1 -> Mux/2
  Q_r,d,x/1 -> Mux/1
  Mux/1 -> Q_r,d/1

== system ctc_sim/inverse kinematics/t -> qt_d/rod 2 ==
  t : Inport
  Mux : Mux  Inputs=2
  Q_r,d,x : Lookup_n-D  NumberOfTableDimensions=1  BreakpointsForDimension1=t_d(1,:)  BreakpointsForDimension2=t_d(1,:)  Table=Q_d((r-1)*2+1,:)  InternalRulePriority=Speed  RndMeth=Simplest  InputSameDT=on
  Q_r,d,y : Lookup_n-D  NumberOfTableDimensions=1  BreakpointsForDimension1=t_d(1,:)  BreakpointsForDimension2=t_d(1,:)  Table=Q_d((r-1)*2+2,:)  InternalRulePriority=Speed  RndMeth=Simplest  InputSameDT=on
  Q_r,d : Outport
  wires:
  t/1 -> Q_r,d,y/1, Q_r,d,x/1
  Q_r,d,y/1 -> Mux/2
  Q_r,d,x/1 -> Mux/1
  Mux/1 -> Q_r,d/1

== system ctc_sim/inverse kinematics/t -> qt_d/rod 3 ==
  t : Inport
  Mux : Mux  Inputs=2
  Q_r,d,x : Lookup_n-D  NumberOfTableDimensions=1  BreakpointsForDimension1=t_d(1,:)  BreakpointsForDimension2=t_d(1,:)  Table=Q_d((r-1)*2+1,:)  InternalRulePriority=Speed  RndMeth=Simplest  InputSameDT=on
  Q_r,d,y : Lookup_n-D  NumberOfTableDimensions=1  BreakpointsForDimension1=t_d(1,:)  BreakpointsForDimension2=t_d(1,:)  Table=Q_d((r-1)*2+2,:)  InternalRulePriority=Speed  RndMeth=Simplest  InputSameDT=on
  Q_r,d : Outport
  wires:
  t/1 -> Q_r,d,y/1, Q_r,d,x/1
  Q_r,d,y/1 -> Mux/2
  Q_r,d,x/1 -> Mux/1
  Mux/1 -> Q_r,d/1

== system ctc_sim/inverse kinematics/t -> qt_d/rod 4 ==
  t : Inport
  Mux : Mux  Inputs=2
  Q_r,d,x : Lookup_n-D  NumberOfTableDimensions=1  BreakpointsForDimension1=t_d(1,:)  BreakpointsForDimension2=t_d(1,:)  Table=Q_d((r-1)*2+1,:)  InternalRulePriority=Speed  RndMeth=Simplest  InputSameDT=on
  Q_r,d,y : Lookup_n-D  NumberOfTableDimensions=1  BreakpointsForDimension1=t_d(1,:)  BreakpointsForDimension2=t_d(1,:)  Table=Q_d((r-1)*2+2,:)  InternalRulePriority=Speed  RndMeth=Simplest  InputSameDT=on
  Q_r,d : Outport
  wires:
  t/1 -> Q_r,d,y/1, Q_r,d,x/1
  Q_r,d,y/1 -> Mux/2
  Q_r,d,x/1 -> Mux/1
  Mux/1 -> Q_r,d/1

== system ctc_sim/inverse kinematics/t -> qt_d/rod 5 ==
  t : Inport
  Mux : Mux  Inputs=2
  Q_r,d,x : Lookup_n-D  NumberOfTableDimensions=1  BreakpointsForDimension1=t_d(1,:)  BreakpointsForDimension2=t_d(1,:)  Table=Q_d((r-1)*2+1,:)  InternalRulePriority=Speed  RndMeth=Simplest  InputSameDT=on
  Q_r,d,y : Lookup_n-D  NumberOfTableDimensions=1  BreakpointsForDimension1=t_d(1,:)  BreakpointsForDimension2=t_d(1,:)  Table=Q_d((r-1)*2+2,:)  InternalRulePriority=Speed  RndMeth=Simplest  InputSameDT=on
  Q_r,d : Outport
  wires:
  t/1 -> Q_r,d,y/1, Q_r,d,x/1
  Q_r,d,y/1 -> Mux/2
  Q_r,d,x/1 -> Mux/1
  Mux/1 -> Q_r,d/1

== system ctc_sim/inverse kinematics/t -> qt_d/rod 6 ==
  t : Inport
  Mux : Mux  Inputs=2
  Q_r,d,x : Lookup_n-D  NumberOfTableDimensions=1  BreakpointsForDimension1=t_d(1,:)  BreakpointsForDimension2=t_d(1,:)  Table=Q_d((r-1)*2+1,:)  InternalRulePriority=Speed  RndMeth=Simplest  InputSameDT=on
  Q_r,d,y : Lookup_n-D  NumberOfTableDimensions=1  BreakpointsForDimension1=t_d(1,:)  BreakpointsForDimension2=t_d(1,:)  Table=Q_d((r-1)*2+2,:)  InternalRulePriority=Speed  RndMeth=Simplest  InputSameDT=on
  Q_r,d : Outport
  wires:
  t/1 -> Q_r,d,y/1, Q_r,d,x/1
  Q_r,d,y/1 -> Mux/2
  Q_r,d,x/1 -> Mux/1
  Mux/1 -> Q_r,d/1

== system ctc_sim/inverse kinematics/t -> qt_d/upper base ==
  t : Inport
  Mux : Mux  Inputs=6
  Q_ub,d,phi_x : Lookup_n-D  NumberOfTableDimensions=1  BreakpointsForDimension1=t_d(1,:)  BreakpointsForDimension2=t_d(1,:)  Table=Q_d(16,:)  InternalRulePriority=Speed  RndMeth=Simplest  InputSameDT=on
  Q_ub,d,phi_y : Lookup_n-D  NumberOfTableDimensions=1  BreakpointsForDimension1=t_d(1,:)  BreakpointsForDimension2=t_d(1,:)  Table=Q_d(17,:)  InternalRulePriority=Speed  RndMeth=Simplest  InputSameDT=on
  Q_ub,d,phi_z : Lookup_n-D  NumberOfTableDimensions=1  BreakpointsForDimension1=t_d(1,:)  BreakpointsForDimension2=t_d(1,:)  Table=Q_d(18,:)  InternalRulePriority=Speed  RndMeth=Simplest  InputSameDT=on
  Q_ub,d,x : Lookup_n-D  NumberOfTableDimensions=1  BreakpointsForDimension1=t_d(1,:)  BreakpointsForDimension2=t_d(1,:)  Table=Q_d(13,:)  InternalRulePriority=Speed  RndMeth=Simplest  InputSameDT=on
  Q_ub,d,y : Lookup_n-D  NumberOfTableDimensions=1  BreakpointsForDimension1=t_d(1,:)  BreakpointsForDimension2=t_d(1,:)  Table=Q_d(14,:)  InternalRulePriority=Speed  RndMeth=Simplest  InputSameDT=on
  Q_ub,d,z : Lookup_n-D  NumberOfTableDimensions=1  BreakpointsForDimension1=t_d(1,:)  BreakpointsForDimension2=t_d(1,:)  Table=Q_d(15,:)  InternalRulePriority=Speed  RndMeth=Simplest  InputSameDT=on
  Q_ub,d : Outport
  wires:
  t/1 -> Q_ub,d,y/1, Q_ub,d,z/1, Q_ub,d,phi_x/1, Q_ub,d,phi_y/1, Q_ub,d,phi_z/1, Q_ub,d,x/1
  Q_ub,d,x/1 -> Mux/1
  Q_ub,d,phi_z/1 -> Mux/6
  Q_ub,d,phi_y/1 -> Mux/5
  Q_ub,d,phi_x/1 -> Mux/4
  Q_ub,d,z/1 -> Mux/3
  Q_ub,d,y/1 -> Mux/2
  Mux/1 -> Q_ub,d/1

== system ctc_sim/inverse kinematics/t -> qtt_d/rod 1 ==
  t : Inport
  Mux : Mux  Inputs=2
  Q_r,d,x : Lookup_n-D  NumberOfTableDimensions=1  BreakpointsForDimension1=t_d(1,:)  BreakpointsForDimension2=t_d(1,:)  Table=Q_d((r-1)*2+1,:)  InternalRulePriority=Speed  RndMeth=Simplest  InputSameDT=on
  Q_r,d,y : Lookup_n-D  NumberOfTableDimensions=1  BreakpointsForDimension1=t_d(1,:)  BreakpointsForDimension2=t_d(1,:)  Table=Q_d((r-1)*2+2,:)  InternalRulePriority=Speed  RndMeth=Simplest  InputSameDT=on
  Q_r,d : Outport
  wires:
  t/1 -> Q_r,d,y/1, Q_r,d,x/1
  Q_r,d,y/1 -> Mux/2
  Q_r,d,x/1 -> Mux/1
  Mux/1 -> Q_r,d/1

== system ctc_sim/inverse kinematics/t -> qtt_d/rod 2 ==
  t : Inport
  Mux : Mux  Inputs=2
  Q_r,d,x : Lookup_n-D  NumberOfTableDimensions=1  BreakpointsForDimension1=t_d(1,:)  BreakpointsForDimension2=t_d(1,:)  Table=Q_d((r-1)*2+1,:)  InternalRulePriority=Speed  RndMeth=Simplest  InputSameDT=on
  Q_r,d,y : Lookup_n-D  NumberOfTableDimensions=1  BreakpointsForDimension1=t_d(1,:)  BreakpointsForDimension2=t_d(1,:)  Table=Q_d((r-1)*2+2,:)  InternalRulePriority=Speed  RndMeth=Simplest  InputSameDT=on
  Q_r,d : Outport
  wires:
  t/1 -> Q_r,d,y/1, Q_r,d,x/1
  Q_r,d,y/1 -> Mux/2
  Q_r,d,x/1 -> Mux/1
  Mux/1 -> Q_r,d/1

== system ctc_sim/inverse kinematics/t -> qtt_d/rod 3 ==
  t : Inport
  Mux : Mux  Inputs=2
  Q_r,d,x : Lookup_n-D  NumberOfTableDimensions=1  BreakpointsForDimension1=t_d(1,:)  BreakpointsForDimension2=t_d(1,:)  Table=Q_d((r-1)*2+1,:)  InternalRulePriority=Speed  RndMeth=Simplest  InputSameDT=on
  Q_r,d,y : Lookup_n-D  NumberOfTableDimensions=1  BreakpointsForDimension1=t_d(1,:)  BreakpointsForDimension2=t_d(1,:)  Table=Q_d((r-1)*2+2,:)  InternalRulePriority=Speed  RndMeth=Simplest  InputSameDT=on
  Q_r,d : Outport
  wires:
  t/1 -> Q_r,d,y/1, Q_r,d,x/1
  Q_r,d,y/1 -> Mux/2
  Q_r,d,x/1 -> Mux/1
  Mux/1 -> Q_r,d/1

== system ctc_sim/inverse kinematics/t -> qtt_d/rod 4 ==
  t : Inport
  Mux : Mux  Inputs=2
  Q_r,d,x : Lookup_n-D  NumberOfTableDimensions=1  BreakpointsForDimension1=t_d(1,:)  BreakpointsForDimension2=t_d(1,:)  Table=Q_d((r-1)*2+1,:)  InternalRulePriority=Speed  RndMeth=Simplest  InputSameDT=on
  Q_r,d,y : Lookup_n-D  NumberOfTableDimensions=1  BreakpointsForDimension1=t_d(1,:)  BreakpointsForDimension2=t_d(1,:)  Table=Q_d((r-1)*2+2,:)  InternalRulePriority=Speed  RndMeth=Simplest  InputSameDT=on
  Q_r,d : Outport
  wires:
  t/1 -> Q_r,d,y/1, Q_r,d,x/1
  Q_r,d,y/1 -> Mux/2
  Q_r,d,x/1 -> Mux/1
  Mux/1 -> Q_r,d/1

== system ctc_sim/inverse kinematics/t -> qtt_d/rod 5 ==
  t : Inport
  Mux : Mux  Inputs=2
  Q_r,d,x : Lookup_n-D  NumberOfTableDimensions=1  BreakpointsForDimension1=t_d(1,:)  BreakpointsForDimension2=t_d(1,:)  Table=Q_d((r-1)*2+1,:)  InternalRulePriority=Speed  RndMeth=Simplest  InputSameDT=on
  Q_r,d,y : Lookup_n-D  NumberOfTableDimensions=1  BreakpointsForDimension1=t_d(1,:)  BreakpointsForDimension2=t_d(1,:)  Table=Q_d((r-1)*2+2,:)  InternalRulePriority=Speed  RndMeth=Simplest  InputSameDT=on
  Q_r,d : Outport
  wires:
  t/1 -> Q_r,d,y/1, Q_r,d,x/1
  Q_r,d,y/1 -> Mux/2
  Q_r,d,x/1 -> Mux/1
  Mux/1 -> Q_r,d/1

== system ctc_sim/inverse kinematics/t -> qtt_d/rod 6 ==
  t : Inport
  Mux : Mux  Inputs=2
  Q_r,d,x : Lookup_n-D  NumberOfTableDimensions=1  BreakpointsForDimension1=t_d(1,:)  BreakpointsForDimension2=t_d(1,:)  Table=Q_d((r-1)*2+1,:)  InternalRulePriority=Speed  RndMeth=Simplest  InputSameDT=on
  Q_r,d,y : Lookup_n-D  NumberOfTableDimensions=1  BreakpointsForDimension1=t_d(1,:)  BreakpointsForDimension2=t_d(1,:)  Table=Q_d((r-1)*2+2,:)  InternalRulePriority=Speed  RndMeth=Simplest  InputSameDT=on
  Q_r,d : Outport
  wires:
  t/1 -> Q_r,d,y/1, Q_r,d,x/1
  Q_r,d,y/1 -> Mux/2
  Q_r,d,x/1 -> Mux/1
  Mux/1 -> Q_r,d/1

== system ctc_sim/inverse kinematics/t -> qtt_d/upper base ==
  t : Inport
  Mux : Mux  Inputs=6
  Q_ub,d,phi_x : Lookup_n-D  NumberOfTableDimensions=1  BreakpointsForDimension1=t_d(1,:)  BreakpointsForDimension2=t_d(1,:)  Table=Q_d(16,:)  InternalRulePriority=Speed  RndMeth=Simplest  InputSameDT=on
  Q_ub,d,phi_y : Lookup_n-D  NumberOfTableDimensions=1  BreakpointsForDimension1=t_d(1,:)  BreakpointsForDimension2=t_d(1,:)  Table=Q_d(17,:)  InternalRulePriority=Speed  RndMeth=Simplest  InputSameDT=on
  Q_ub,d,phi_z : Lookup_n-D  NumberOfTableDimensions=1  BreakpointsForDimension1=t_d(1,:)  BreakpointsForDimension2=t_d(1,:)  Table=Q_d(18,:)  InternalRulePriority=Speed  RndMeth=Simplest  InputSameDT=on
  Q_ub,d,x : Lookup_n-D  NumberOfTableDimensions=1  BreakpointsForDimension1=t_d(1,:)  BreakpointsForDimension2=t_d(1,:)  Table=Q_d(13,:)  InternalRulePriority=Speed  RndMeth=Simplest  InputSameDT=on
  Q_ub,d,y : Lookup_n-D  NumberOfTableDimensions=1  BreakpointsForDimension1=t_d(1,:)  BreakpointsForDimension2=t_d(1,:)  Table=Q_d(14,:)  InternalRulePriority=Speed  RndMeth=Simplest  InputSameDT=on
  Q_ub,d,z : Lookup_n-D  NumberOfTableDimensions=1  BreakpointsForDimension1=t_d(1,:)  BreakpointsForDimension2=t_d(1,:)  Table=Q_d(15,:)  InternalRulePriority=Speed  RndMeth=Simplest  InputSameDT=on
  Q_ub,d : Outport
  wires:
  t/1 -> Q_ub,d,y/1, Q_ub,d,z/1, Q_ub,d,phi_x/1, Q_ub,d,phi_y/1, Q_ub,d,phi_z/1, Q_ub,d,x/1
  Q_ub,d,x/1 -> Mux/1
  Q_ub,d,phi_z/1 -> Mux/6
  Q_ub,d,phi_y/1 -> Mux/5
  Q_ub,d,phi_x/1 -> Mux/4
  Q_ub,d,z/1 -> Mux/3
  Q_ub,d,y/1 -> Mux/2
  Mux/1 -> Q_ub,d/1

== system ctc_sim/computed torgue control/bases + rods/lower base/O_lb -> G_1 ==
  rot z : sm_lib/Frames and Transforms/Rigid Transform  TranslationMethod=None  TranslationStandardOffset=0  TranslationLengthUnit=m  TranslationStandardAxis=+Z  TranslationCartesianOffset=[0 0 0]  TranslationROffset=0  TranslationROffsetUnits=m  TranslationZOffset=0  TranslationZOffsetUnits=m  TranslationThetaOffset=0  TranslationThetaOffsetUnits=deg  RotationMethod=StandardAxis  RotationAngleUnits=rad  RotationStandardAxis=+Z  RotationAngle=Fi_b_z(1)  RotationArbitraryAxis=[0 0 1]  FollAlignAxisA=+X  BaseAlignAxisA=+Y  FollAlignAxisB=+Y  BaseAlignAxisB=+Z  RotationSequenceAxes=FollowerAxes  RotationSequence=XYX  RotationSequenceAngles=[0 0 0]  RotationSequenceAnglesUnits=deg  RotationMatrix=[1 0 0; 0 1 0; 0 0 1]
  trans z : sm_lib/Frames and Transforms/Rigid Transform  TranslationMethod=StandardAxis  TranslationStandardOffset=h_lb  TranslationLengthUnit=m  TranslationStandardAxis=+Z  TranslationCartesianOffset=[0 0 0]  TranslationROffset=0  TranslationROffsetUnits=m  TranslationZOffset=0  TranslationZOffsetUnits=m  TranslationThetaOffset=0  TranslationThetaOffsetUnits=deg  RotationMethod=None  RotationAngleUnits=deg  RotationStandardAxis=+Z  RotationAngle=0.0  RotationArbitraryAxis=[0 0 1]  FollAlignAxisA=+X  BaseAlignAxisA=+Y  FollAlignAxisB=+Y  BaseAlignAxisB=+Z  RotationSequenceAxes=FollowerAxes  RotationSequence=XYX  RotationSequenceAngles=[0 0 0]  RotationSequenceAnglesUnits=deg  RotationMatrix=[1 0 0; 0 1 0; 0 0 1]
  transl y : sm_lib/Frames and Transforms/Rigid Transform  TranslationMethod=StandardAxis  TranslationStandardOffset=w_lb/2  TranslationLengthUnit=m  TranslationStandardAxis=+Y  TranslationCartesianOffset=[0 0 0]  TranslationROffset=0  TranslationROffsetUnits=m  TranslationZOffset=0  TranslationZOffsetUnits=m  TranslationThetaOffset=0  TranslationThetaOffsetUnits=deg  RotationMethod=None  RotationAngleUnits=deg  RotationStandardAxis=+Z  RotationAngle=0.0  RotationArbitraryAxis=[0 0 1]  FollAlignAxisA=+X  BaseAlignAxisA=+Y  FollAlignAxisB=+Y  BaseAlignAxisB=+Z  RotationSequenceAxes=FollowerAxes  RotationSequence=XYX  RotationSequenceAngles=[0 0 0]  RotationSequenceAnglesUnits=deg  RotationMatrix=[1 0 0; 0 1 0; 0 0 1]
  O_lb : PMIOPort  Side=Left
  G_1 : PMIOPort  Port=2  Side=Right
  connections:
  trans z/LConn1 -- O_lb/RConn1
  trans z/RConn1 -- rot z/LConn1
  transl y/LConn1 -- rot z/RConn1
  transl y/RConn1 -- G_1/RConn1
